simulink model "FSAC2021_V1"  (R2014a)
settings: Solver=FixedStepDiscrete  StartTime=0.0  StopTime=inf  FixedStep=0.0005  RelTol=1e-3
model workspace (MAT data in the model file):
  MCOS : class17 (value not decoded)
  MCOS : class17 (value not decoded)
  MCOS : class17 (value not decoded)
  MCOS : class17 (value not decoded)
  MCOS : class17 (value not decoded)
  MCOS : class17 (value not decoded)
  MCOS : class17 (value not decoded)
  MCOS : class17 (value not decoded)
  MCOS : class17 (value not decoded)
  MCOS : class17 (value not decoded)
  MCOS : class17 (value not decoded)
  MCOS : class17 (value not decoded)
  MCOS : class17 (value not decoded)
  MCOS : class17 (value not decoded)
  MCOS : class17 (value not decoded)
  MCOS : class17 (value not decoded)
  MCOS : class17 (value not decoded)
  MCOS : class17 (value not decoded)
  MCOS : class17 (value not decoded)
  BUZZER_START = 1
  MCOS : class17 (value not decoded)
  MCOS : class17 (value not decoded)
  MCOS : class17 (value not decoded)
  MCOS : class17 (value not decoded)
  MCOS : class17 (value not decoded)
  MCOS : class17 (value not decoded)
  MCOS : class17 (value not decoded)
  MCOS : class17 (value not decoded)
  MCOS : class17 (value not decoded)
  MCOS : class17 (value not decoded)
  MCOS : class17 (value not decoded)
  MCOS : class17 (value not decoded)
  MCOS : class17 (value not decoded)
  MCOS : class17 (value not decoded)
  MCOS : class17 (value not decoded)
  MCOS : class17 (value not decoded)
  MCOS : class17 (value not decoded)
  MCOS : class17 (value not decoded)
  MCOS : class17 (value not decoded)
  MCOS : class17 (value not decoded)
  MCOS : class17 (value not decoded)
  MCOS : class17 (value not decoded)
  MCOS : class17 (value not decoded)
  MCOS : class17 (value not decoded)
  MCOS : class17 (value not decoded)
  MCOS : class17 (value not decoded)
  MCOS : class17 (value not decoded)
  MCOS : class17 (value not decoded)
  MCOS : class17 (value not decoded)
  MCOS : class17 (value not decoded)
  MCOS : class17 (value not decoded)
  MCOS : class17 (value not decoded)
  MCOS : class17 (value not decoded)
  MCOS : class17 (value not decoded)
  MCOS : class17 (value not decoded)
  MCOS : class17 (value not decoded)
  MCOS : class17 (value not decoded)
  MCOS : class17 (value not decoded)
  Brake = 11
  MCOS : class17 (value not decoded)
  MCOS : class17 (value not decoded)
  MCOS : class17 (value not decoded)
  MCOS : class17 (value not decoded)
  MCOS : class17 (value not decoded)
  MCOS : class17 (value not decoded)
  MCOS : class17 (value not decoded)
  MCOS : class17 (value not decoded)
  Sensor_Acc_b = 101.85
  Sensor_Acc_k = -0.0185
  Str_Sen_Orig_Angle = -341
  MCOS : class17 (value not decoded)
  Tire_D = 0.47
  T = 0.05
libraries: simulink x189, ec55xxlib x135
(part 7 of 9)

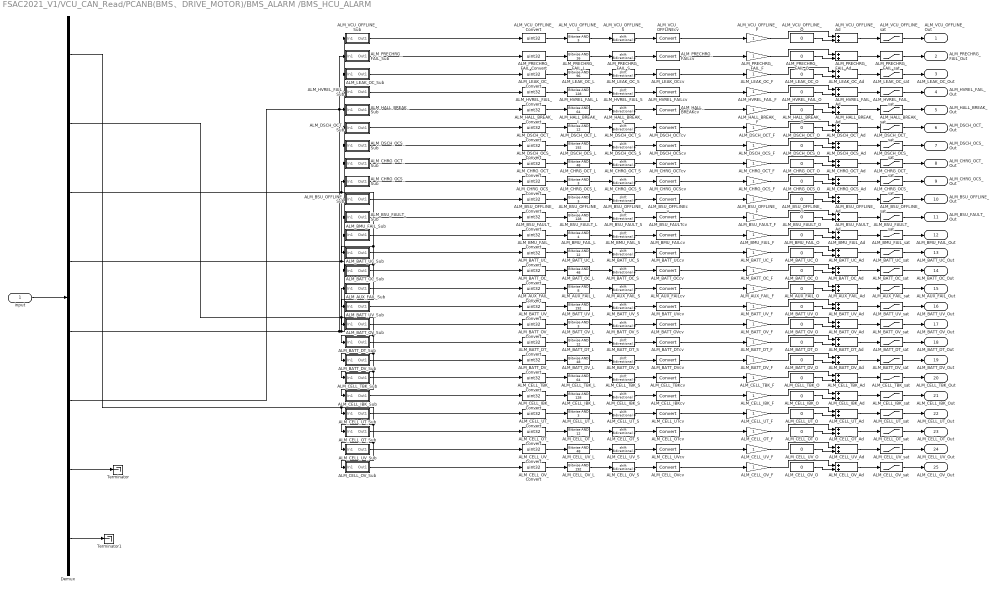
== system FSAC2021_V1/VCU_CAN_Read/PCANB(BMS、DRIVE_MOTOR)/BMS_ALARM /BMS_HCU_ALARM ==
  input : Inport
  ALM_AUX_FAIL_Ad : Sum
  ALM_AUX_FAIL_Convert : DataTypeConversion  OutDataTypeStr=uint32
  ALM_AUX_FAIL_F : Gain
  ALM_AUX_FAIL_L : simulink/Logic and Bit Operations/Bitwise Operator  logicop=AND  UseBitMask=on  BitMask=8  BitMaskRealWorld=Stored Integer
  ALM_AUX_FAIL_O : Constant  Value=0  OutDataTypeStr=single
  ALM_AUX_FAIL_S : ArithShift  BitShiftNumber=3
  ALM_AUX_FAIL_Sub : Subsystem
  ALM_AUX_FAIL_sat : Saturate  UpperLimit=1  LowerLimit=0
  ALM_AUX_FAILcv : DataTypeConversion
  ALM_BATT_DT_Ad : Sum
  ALM_BATT_DT_Convert : DataTypeConversion  OutDataTypeStr=uint32
  ALM_BATT_DT_F : Gain
  ALM_BATT_DT_L : simulink/Logic and Bit Operations/Bitwise Operator  logicop=AND  UseBitMask=on  BitMask=12  BitMaskRealWorld=Stored Integer
  ALM_BATT_DT_O : Constant  Value=0  OutDataTypeStr=single
  ALM_BATT_DT_S : ArithShift  BitShiftNumber=2
  ALM_BATT_DT_Sub : Subsystem
  ALM_BATT_DT_sat : Saturate  UpperLimit=3  LowerLimit=0
  ALM_BATT_DTcv : DataTypeConversion
  ALM_BATT_DV_Ad : Sum
  ALM_BATT_DV_Convert : DataTypeConversion  OutDataTypeStr=uint32
  ALM_BATT_DV_F : Gain
  ALM_BATT_DV_L : simulink/Logic and Bit Operations/Bitwise Operator  logicop=AND  UseBitMask=on  BitMask=48  BitMaskRealWorld=Stored Integer
  ALM_BATT_DV_O : Constant  Value=0  OutDataTypeStr=single
  ALM_BATT_DV_S : ArithShift  BitShiftNumber=4
  ALM_BATT_DV_Sub : Subsystem
  ALM_BATT_DV_sat : Saturate  UpperLimit=3  LowerLimit=0
  ALM_BATT_DVcv : DataTypeConversion
  ALM_BATT_OC_Ad : Sum
  ALM_BATT_OC_Convert : DataTypeConversion  OutDataTypeStr=uint32
  ALM_BATT_OC_F : Gain
  ALM_BATT_OC_L : simulink/Logic and Bit Operations/Bitwise Operator  logicop=AND  UseBitMask=on  BitMask=48  BitMaskRealWorld=Stored Integer
  ALM_BATT_OC_O : Constant  Value=0  OutDataTypeStr=single
  ALM_BATT_OC_S : ArithShift  BitShiftNumber=4
  ALM_BATT_OC_Sub : Subsystem
  ALM_BATT_OC_sat : Saturate  UpperLimit=3  LowerLimit=0
  ALM_BATT_OCcv : DataTypeConversion
  ALM_BATT_OV_Ad : Sum
  ALM_BATT_OV_Convert : DataTypeConversion  OutDataTypeStr=uint32
  ALM_BATT_OV_F : Gain
  ALM_BATT_OV_L : simulink/Logic and Bit Operations/Bitwise Operator  logicop=AND  UseBitMask=on  BitMask=3  BitMaskRealWorld=Stored Integer
  ALM_BATT_OV_O : Constant  Value=0  OutDataTypeStr=single
  ALM_BATT_OV_S : ArithShift
  ALM_BATT_OV_Sub : Subsystem
  ALM_BATT_OV_sat : Saturate  UpperLimit=3  LowerLimit=0
  ALM_BATT_OVcv : DataTypeConversion
  ALM_BATT_UC_Ad : Sum
  ALM_BATT_UC_Convert : DataTypeConversion  OutDataTypeStr=uint32
  ALM_BATT_UC_F : Gain
  ALM_BATT_UC_L : simulink/Logic and Bit Operations/Bitwise Operator  logicop=AND  UseBitMask=on  BitMask=12  BitMaskRealWorld=Stored Integer
  ALM_BATT_UC_O : Constant  Value=0  OutDataTypeStr=single
  ALM_BATT_UC_S : ArithShift  BitShiftNumber=2
  ALM_BATT_UC_Sub : Subsystem
  ALM_BATT_UC_sat : Saturate  UpperLimit=3  LowerLimit=0
  ALM_BATT_UCcv : DataTypeConversion
  ALM_BATT_UV_Ad : Sum
  ALM_BATT_UV_Convert : DataTypeConversion  OutDataTypeStr=uint32
  ALM_BATT_UV_F : Gain
  ALM_BATT_UV_L : simulink/Logic and Bit Operations/Bitwise Operator  logicop=AND  UseBitMask=on  BitMask=192  BitMaskRealWorld=Stored Integer
  ALM_BATT_UV_O : Constant  Value=0  OutDataTypeStr=single
  ALM_BATT_UV_S : ArithShift  BitShiftNumber=6
  ALM_BATT_UV_Sub : Subsystem
  ALM_BATT_UV_sat : Saturate  UpperLimit=3  LowerLimit=0
  ALM_BATT_UVcv : DataTypeConversion
  ALM_BMU_FAIL_Ad : Sum
  ALM_BMU_FAIL_Convert : DataTypeConversion  OutDataTypeStr=uint32
  ALM_BMU_FAIL_F : Gain
  ALM_BMU_FAIL_L : simulink/Logic and Bit Operations/Bitwise Operator  logicop=AND  UseBitMask=on  BitMask=4  BitMaskRealWorld=Stored Integer
  ALM_BMU_FAIL_O : Constant  Value=0  OutDataTypeStr=single
  ALM_BMU_FAIL_S : ArithShift  BitShiftNumber=2
  ALM_BMU_FAIL_Sub : Subsystem
  ALM_BMU_FAIL_sat : Saturate  UpperLimit=1  LowerLimit=0
  ALM_BMU_FAILcv : DataTypeConversion
  ALM_BSU_FAULT_Ad : Sum
  ALM_BSU_FAULT_Convert : DataTypeConversion  OutDataTypeStr=uint32
  ALM_BSU_FAULT_F : Gain
  ALM_BSU_FAULT_L : simulink/Logic and Bit Operations/Bitwise Operator  logicop=AND  UseBitMask=on  BitMask=128  BitMaskRealWorld=Stored Integer
  ALM_BSU_FAULT_O : Constant  Value=0  OutDataTypeStr=single
  ALM_BSU_FAULT_S : ArithShift  BitShiftNumber=7
  ALM_BSU_FAULT_Sub : Subsystem
  ALM_BSU_FAULT_sat : Saturate  UpperLimit=1  LowerLimit=0
  ALM_BSU_FAULTcv : DataTypeConversion
  ALM_BSU_OFFLINE_Ad : Sum
  ALM_BSU_OFFLINE_Convert : DataTypeConversion  OutDataTypeStr=uint32
  ALM_BSU_OFFLINE_F : Gain
  ALM_BSU_OFFLINE_L : simulink/Logic and Bit Operations/Bitwise Operator  logicop=AND  UseBitMask=on  BitMask=3  BitMaskRealWorld=Stored Integer
  ALM_BSU_OFFLINE_O : Constant  Value=0  OutDataTypeStr=single
  ALM_BSU_OFFLINE_S : ArithShift
  ALM_BSU_OFFLINE_Sub : Subsystem
  ALM_BSU_OFFLINE_sat : Saturate  UpperLimit=3  LowerLimit=0
  ALM_BSU_OFFLINEcv : DataTypeConversion
  ALM_CELL_IBK_Ad : Sum
  ALM_CELL_IBK_Convert : DataTypeConversion  OutDataTypeStr=uint32
  ALM_CELL_IBK_F : Gain
  ALM_CELL_IBK_L : simulink/Logic and Bit Operations/Bitwise Operator  logicop=AND  UseBitMask=on  BitMask=128  BitMaskRealWorld=Stored Integer
  ALM_CELL_IBK_O : Constant  Value=0  OutDataTypeStr=single
  ALM_CELL_IBK_S : ArithShift  BitShiftNumber=7
  ALM_CELL_IBK_Sub : Subsystem
  ALM_CELL_IBK_sat : Saturate  UpperLimit=1  LowerLimit=0
  ALM_CELL_IBKcv : DataTypeConversion
  ALM_CELL_OT_Ad : Sum
  ALM_CELL_OT_Convert : DataTypeConversion  OutDataTypeStr=uint32
  ALM_CELL_OT_F : Gain
  ALM_CELL_OT_L : simulink/Logic and Bit Operations/Bitwise Operator  logicop=AND  UseBitMask=on  BitMask=12  BitMaskRealWorld=Stored Integer
  ALM_CELL_OT_O : Constant  Value=0  OutDataTypeStr=single
  ALM_CELL_OT_S : ArithShift  BitShiftNumber=2
  ALM_CELL_OT_Sub : Subsystem
  ALM_CELL_OT_sat : Saturate  UpperLimit=3  LowerLimit=0
  ALM_CELL_OTcv : DataTypeConversion
  ALM_CELL_OV_Ad : Sum
  ALM_CELL_OV_Convert : DataTypeConversion  OutDataTypeStr=uint32
  ALM_CELL_OV_F : Gain
  ALM_CELL_OV_L : simulink/Logic and Bit Operations/Bitwise Operator  logicop=AND  UseBitMask=on  BitMask=192  BitMaskRealWorld=Stored Integer
  ALM_CELL_OV_O : Constant  Value=0  OutDataTypeStr=single
  ALM_CELL_OV_S : ArithShift  BitShiftNumber=6
  ALM_CELL_OV_Sub : Subsystem
  ALM_CELL_OV_sat : Saturate  UpperLimit=3  LowerLimit=0
  ALM_CELL_OVcv : DataTypeConversion
  ALM_CELL_TBK_Ad : Sum
  ALM_CELL_TBK_Convert : DataTypeConversion  OutDataTypeStr=uint32
  ALM_CELL_TBK_F : Gain
  ALM_CELL_TBK_L : simulink/Logic and Bit Operations/Bitwise Operator  logicop=AND  UseBitMask=on  BitMask=64  BitMaskRealWorld=Stored Integer
  ALM_CELL_TBK_O : Constant  Value=0  OutDataTypeStr=single
  ALM_CELL_TBK_S : ArithShift  BitShiftNumber=6
  ALM_CELL_TBK_Sub : Subsystem
  ALM_CELL_TBK_sat : Saturate  UpperLimit=1  LowerLimit=0
  ALM_CELL_TBKcv : DataTypeConversion
  ALM_CELL_UT_Ad : Sum
  ALM_CELL_UT_Convert : DataTypeConversion  OutDataTypeStr=uint32
  ALM_CELL_UT_F : Gain
  ALM_CELL_UT_L : simulink/Logic and Bit Operations/Bitwise Operator  logicop=AND  UseBitMask=on  BitMask=3  BitMaskRealWorld=Stored Integer
  ALM_CELL_UT_O : Constant  Value=0  OutDataTypeStr=single
  ALM_CELL_UT_S : ArithShift
  ALM_CELL_UT_Sub : Subsystem
  ALM_CELL_UT_sat : Saturate  UpperLimit=3  LowerLimit=0
  ALM_CELL_UTcv : DataTypeConversion
  ALM_CELL_UV_Ad : Sum
  ALM_CELL_UV_Convert : DataTypeConversion  OutDataTypeStr=uint32
  ALM_CELL_UV_F : Gain
  ALM_CELL_UV_L : simulink/Logic and Bit Operations/Bitwise Operator  logicop=AND  UseBitMask=on  BitMask=48  BitMaskRealWorld=Stored Integer
  ALM_CELL_UV_O : Constant  Value=0  OutDataTypeStr=single
  ALM_CELL_UV_S : ArithShift  BitShiftNumber=4
  ALM_CELL_UV_Sub : Subsystem
  ALM_CELL_UV_sat : Saturate  UpperLimit=3  LowerLimit=0
  ALM_CELL_UVcv : DataTypeConversion
  ALM_CHRG_OCS_Ad : Sum
  ALM_CHRG_OCS_Convert : DataTypeConversion  OutDataTypeStr=uint32
  ALM_CHRG_OCS_F : Gain
  ALM_CHRG_OCS_L : simulink/Logic and Bit Operations/Bitwise Operator  logicop=AND  UseBitMask=on  BitMask=3  BitMaskRealWorld=Stored Integer
  ALM_CHRG_OCS_O : Constant  Value=0  OutDataTypeStr=single
  ALM_CHRG_OCS_S : ArithShift
  ALM_CHRG_OCS_Sub : Subsystem
  ALM_CHRG_OCS_sat : Saturate  UpperLimit=3  LowerLimit=0
  ALM_CHRG_OCScv : DataTypeConversion
  ALM_CHRG_OCT_Ad : Sum
  ALM_CHRG_OCT_Convert : DataTypeConversion  OutDataTypeStr=uint32
  ALM_CHRG_OCT_F : Gain
  ALM_CHRG_OCT_L : simulink/Logic and Bit Operations/Bitwise Operator  logicop=AND  UseBitMask=on  BitMask=48  BitMaskRealWorld=Stored Integer
  ALM_CHRG_OCT_O : Constant  Value=0  OutDataTypeStr=single
  ALM_CHRG_OCT_S : ArithShift  BitShiftNumber=4
  ALM_CHRG_OCT_Sub : Subsystem
  ALM_CHRG_OCT_sat : Saturate  UpperLimit=3  LowerLimit=0
  ALM_CHRG_OCTcv : DataTypeConversion
  ALM_DSCH_OCS_Ad : Sum
  ALM_DSCH_OCS_Convert : DataTypeConversion  OutDataTypeStr=uint32
  ALM_DSCH_OCS_F : Gain
  ALM_DSCH_OCS_L : simulink/Logic and Bit Operations/Bitwise Operator  logicop=AND  UseBitMask=on  BitMask=192  BitMaskRealWorld=Stored Integer
  ALM_DSCH_OCS_O : Constant  Value=0  OutDataTypeStr=single
  ALM_DSCH_OCS_S : ArithShift  BitShiftNumber=6
  ALM_DSCH_OCS_Sub : Subsystem
  ALM_DSCH_OCS_sat : Saturate  UpperLimit=3  LowerLimit=0
  ALM_DSCH_OCScv : DataTypeConversion
  ALM_DSCH_OCT_Ad : Sum
  ALM_DSCH_OCT_Convert : DataTypeConversion  OutDataTypeStr=uint32
  ALM_DSCH_OCT_F : Gain
  ALM_DSCH_OCT_L : simulink/Logic and Bit Operations/Bitwise Operator  logicop=AND  UseBitMask=on  BitMask=12  BitMaskRealWorld=Stored Integer
  ALM_DSCH_OCT_O : Constant  Value=0  OutDataTypeStr=single
  ALM_DSCH_OCT_S : ArithShift  BitShiftNumber=2
  ALM_DSCH_OCT_Sub : Subsystem
  ALM_DSCH_OCT_sat : Saturate  UpperLimit=3  LowerLimit=0
  ALM_DSCH_OCTcv : DataTypeConversion
  ALM_HALL_BREAK_Ad : Sum
  ALM_HALL_BREAK_Convert : DataTypeConversion  OutDataTypeStr=uint32
  ALM_HALL_BREAK_F : Gain
  ALM_HALL_BREAK_L : simulink/Logic and Bit Operations/Bitwise Operator  logicop=AND  UseBitMask=on  BitMask=64  BitMaskRealWorld=Stored Integer
  ALM_HALL_BREAK_O : Constant  Value=0  OutDataTypeStr=single
  ALM_HALL_BREAK_S : ArithShift  BitShiftNumber=6
  ALM_HALL_BREAK_Sub : Subsystem
  ALM_HALL_BREAK_sat : Saturate  UpperLimit=1  LowerLimit=0
  ALM_HALL_BREAKcv : DataTypeConversion
  ALM_HVREL_FAIL_Ad : Sum
  ALM_HVREL_FAIL_Convert : DataTypeConversion  OutDataTypeStr=uint32
  ALM_HVREL_FAIL_F : Gain
  ALM_HVREL_FAIL_L : simulink/Logic and Bit Operations/Bitwise Operator  logicop=AND  UseBitMask=on  BitMask=128  BitMaskRealWorld=Stored Integer
  ALM_HVREL_FAIL_O : Constant  Value=0  OutDataTypeStr=single
  ALM_HVREL_FAIL_S : ArithShift  BitShiftNumber=7
  ALM_HVREL_FAIL_Sub : Subsystem
  ALM_HVREL_FAIL_sat : Saturate  UpperLimit=1  LowerLimit=0
  ALM_HVREL_FAILcv : DataTypeConversion
  ALM_LEAK_OC_Ad : Sum
  ALM_LEAK_OC_Convert : DataTypeConversion  OutDataTypeStr=uint32
  ALM_LEAK_OC_F : Gain
  ALM_LEAK_OC_L : simulink/Logic and Bit Operations/Bitwise Operator  logicop=AND  UseBitMask=on  BitMask=96  BitMaskRealWorld=Stored Integer
  ALM_LEAK_OC_O : Constant  Value=0  OutDataTypeStr=single
  ALM_LEAK_OC_S : ArithShift  BitShiftNumber=5
  ALM_LEAK_OC_Sub : Subsystem
  ALM_LEAK_OC_sat : Saturate  UpperLimit=3  LowerLimit=0
  ALM_LEAK_OCcv : DataTypeConversion
  ALM_PRECHRG_FAIL_Ad : Sum
  ALM_PRECHRG_FAIL_Convert : DataTypeConversion  OutDataTypeStr=uint32
  ALM_PRECHRG_FAIL_F : Gain
  ALM_PRECHRG_FAIL_L : simulink/Logic and Bit Operations/Bitwise Operator  logicop=AND  UseBitMask=on  BitMask=16  BitMaskRealWorld=Stored Integer
  ALM_PRECHRG_FAIL_O : Constant  Value=0  OutDataTypeStr=single
  ALM_PRECHRG_FAIL_S : ArithShift  BitShiftNumber=4
  ALM_PRECHRG_FAIL_Sub : Subsystem
  ALM_PRECHRG_FAIL_sat : Saturate  UpperLimit=1  LowerLimit=0
  ALM_PRECHRG_FAILcv : DataTypeConversion
  ALM_VCU_OFFLINE_Ad : Sum
  ALM_VCU_OFFLINE_Convert : DataTypeConversion  OutDataTypeStr=uint32
  ALM_VCU_OFFLINE_F : Gain
  ALM_VCU_OFFLINE_L : simulink/Logic and Bit Operations/Bitwise Operator  logicop=AND  UseBitMask=on  BitMask=3  BitMaskRealWorld=Stored Integer
  ALM_VCU_OFFLINE_O : Constant  Value=0  OutDataTypeStr=single
  ALM_VCU_OFFLINE_S : ArithShift
  ALM_VCU_OFFLINE_Sub : Subsystem
  ALM_VCU_OFFLINE_sat : Saturate  UpperLimit=3  LowerLimit=0
  ALM_VCU_OFFLINEcv : DataTypeConversion
  Demux : Demux  Outputs=8
  Terminator : Terminator
  Terminator1 : Terminator
  ALM_VCU_OFFLINE_Out : Outport
  ALM_PRECHRG_FAIL_Out : Outport  Port=2
  ALM_LEAK_OC_Out : Outport  Port=3
  ALM_HVREL_FAIL_Out : Outport  Port=4
  ALM_HALL_BREAK_Out : Outport  Port=5
  ALM_DSCH_OCT_Out : Outport  Port=6
  ALM_DSCH_OCS_Out : Outport  Port=7
  ALM_CHRG_OCT_Out : Outport  Port=8
  ALM_CHRG_OCS_Out : Outport  Port=9
  ALM_BSU_OFFLINE_Out : Outport  Port=10
  ALM_BSU_FAULT_Out : Outport  Port=11
  ALM_BMU_FAIL_Out : Outport  Port=12
  ALM_BATT_UC_Out : Outport  Port=13
  ALM_BATT_OC_Out : Outport  Port=14
  ALM_AUX_FAIL_Out : Outport  Port=15
  ALM_BATT_UV_Out : Outport  Port=16
  ALM_BATT_OV_Out : Outport  Port=17
  ALM_BATT_DT_Out : Outport  Port=18
  ALM_BATT_DV_Out : Outport  Port=19
  ALM_CELL_TBK_Out : Outport  Port=20
  ALM_CELL_IBK_Out : Outport  Port=21
  ALM_CELL_UT_Out : Outport  Port=22
  ALM_CELL_OT_Out : Outport  Port=23
  ALM_CELL_UV_Out : Outport  Port=24
  ALM_CELL_OV_Out : Outport  Port=25
  wires:
  ALM_VCU_OFFLINE_F/1 -> ALM_VCU_OFFLINE_Ad/1
  ALM_VCU_OFFLINE_O/1 -> ALM_VCU_OFFLINE_Ad/2
  ALM_VCU_OFFLINE_Ad/1 -> ALM_VCU_OFFLINE_sat/1
  ALM_VCU_OFFLINE_sat/1 -> ALM_VCU_OFFLINE_Out/1
  Demux/5 -> ALM_VCU_OFFLINE_Sub/1(In1), ALM_LEAK_OC_Sub/1(In1), ALM_BSU_FAULT_Sub/1(In1), ALM_BMU_FAIL_Sub/1(In1), ALM_AUX_FAIL_Sub/1(In1), ALM_PRECHRG_FAIL_Sub/1(In1)
  ALM_VCU_OFFLINE_Sub/1(Out1) -> ALM_VCU_OFFLINE_Convert/1
  ALM_VCU_OFFLINE_Convert/1 -> ALM_VCU_OFFLINE_L/1
  ALM_VCU_OFFLINE_L/1 -> ALM_VCU_OFFLINE_S/1
  ALM_VCU_OFFLINE_S/1 -> ALM_VCU_OFFLINEcv/1
  ALM_VCU_OFFLINEcv/1 -> ALM_VCU_OFFLINE_F/1
  ALM_PRECHRG_FAIL_F/1 -> ALM_PRECHRG_FAIL_Ad/1
  ALM_PRECHRG_FAIL_O/1 -> ALM_PRECHRG_FAIL_Ad/2
  ALM_PRECHRG_FAIL_Ad/1 -> ALM_PRECHRG_FAIL_sat/1
  ALM_PRECHRG_FAIL_sat/1 -> ALM_PRECHRG_FAIL_Out/1
  ALM_PRECHRG_FAIL_Sub/1(Out1) -> ALM_PRECHRG_FAIL_Convert/1
  ALM_PRECHRG_FAIL_Convert/1 -> ALM_PRECHRG_FAIL_L/1
  ALM_PRECHRG_FAIL_L/1 -> ALM_PRECHRG_FAIL_S/1
  ALM_PRECHRG_FAIL_S/1 -> ALM_PRECHRG_FAILcv/1
  ALM_PRECHRG_FAILcv/1 -> ALM_PRECHRG_FAIL_F/1
  ALM_LEAK_OC_F/1 -> ALM_LEAK_OC_Ad/1
  ALM_LEAK_OC_O/1 -> ALM_LEAK_OC_Ad/2
  ALM_LEAK_OC_Ad/1 -> ALM_LEAK_OC_sat/1
  ALM_LEAK_OC_sat/1 -> ALM_LEAK_OC_Out/1
  ALM_LEAK_OC_Sub/1(Out1) -> ALM_LEAK_OC_Convert/1
  ALM_LEAK_OC_Convert/1 -> ALM_LEAK_OC_L/1
  ALM_LEAK_OC_L/1 -> ALM_LEAK_OC_S/1
  ALM_LEAK_OC_S/1 -> ALM_LEAK_OCcv/1
  ALM_LEAK_OCcv/1 -> ALM_LEAK_OC_F/1
  ALM_HVREL_FAIL_F/1 -> ALM_HVREL_FAIL_Ad/1
  ALM_HVREL_FAIL_O/1 -> ALM_HVREL_FAIL_Ad/2
  ALM_HVREL_FAIL_Ad/1 -> ALM_HVREL_FAIL_sat/1
  ALM_HVREL_FAIL_sat/1 -> ALM_HVREL_FAIL_Out/1
  Demux/6 -> ALM_HVREL_FAIL_Sub/1(In1), ALM_HALL_BREAK_Sub/1(In1)
  ALM_HVREL_FAIL_Sub/1(Out1) -> ALM_HVREL_FAIL_Convert/1
  ALM_HVREL_FAIL_Convert/1 -> ALM_HVREL_FAIL_L/1
  ALM_HVREL_FAIL_L/1 -> ALM_HVREL_FAIL_S/1
  ALM_HVREL_FAIL_S/1 -> ALM_HVREL_FAILcv/1
  ALM_HVREL_FAILcv/1 -> ALM_HVREL_FAIL_F/1
  ALM_HALL_BREAK_F/1 -> ALM_HALL_BREAK_Ad/1
  ALM_HALL_BREAK_O/1 -> ALM_HALL_BREAK_Ad/2
  ALM_HALL_BREAK_Ad/1 -> ALM_HALL_BREAK_sat/1
  ALM_HALL_BREAK_sat/1 -> ALM_HALL_BREAK_Out/1
  ALM_HALL_BREAK_Sub/1(Out1) -> ALM_HALL_BREAK_Convert/1
  ALM_HALL_BREAK_Convert/1 -> ALM_HALL_BREAK_L/1
  ALM_HALL_BREAK_L/1 -> ALM_HALL_BREAK_S/1
  ALM_HALL_BREAK_S/1 -> ALM_HALL_BREAKcv/1
  ALM_HALL_BREAKcv/1 -> ALM_HALL_BREAK_F/1
  ALM_DSCH_OCT_F/1 -> ALM_DSCH_OCT_Ad/1
  ALM_DSCH_OCT_O/1 -> ALM_DSCH_OCT_Ad/2
  ALM_DSCH_OCT_Ad/1 -> ALM_DSCH_OCT_sat/1
  ALM_DSCH_OCT_sat/1 -> ALM_DSCH_OCT_Out/1
  Demux/4 -> ALM_DSCH_OCT_Sub/1(In1), ALM_DSCH_OCS_Sub/1(In1), ALM_CHRG_OCT_Sub/1(In1), ALM_BSU_OFFLINE_Sub/1(In1)
  ALM_DSCH_OCT_Sub/1(Out1) -> ALM_DSCH_OCT_Convert/1
  ALM_DSCH_OCT_Convert/1 -> ALM_DSCH_OCT_L/1
  ALM_DSCH_OCT_L/1 -> ALM_DSCH_OCT_S/1
  ALM_DSCH_OCT_S/1 -> ALM_DSCH_OCTcv/1
  ALM_DSCH_OCTcv/1 -> ALM_DSCH_OCT_F/1
  ALM_DSCH_OCS_F/1 -> ALM_DSCH_OCS_Ad/1
  ALM_DSCH_OCS_O/1 -> ALM_DSCH_OCS_Ad/2
  ALM_DSCH_OCS_Ad/1 -> ALM_DSCH_OCS_sat/1
  ALM_DSCH_OCS_sat/1 -> ALM_DSCH_OCS_Out/1
  ALM_DSCH_OCS_Sub/1(Out1) -> ALM_DSCH_OCS_Convert/1
  ALM_DSCH_OCS_Convert/1 -> ALM_DSCH_OCS_L/1
  ALM_DSCH_OCS_L/1 -> ALM_DSCH_OCS_S/1
  ALM_DSCH_OCS_S/1 -> ALM_DSCH_OCScv/1
  ALM_DSCH_OCScv/1 -> ALM_DSCH_OCS_F/1
  ALM_CHRG_OCT_F/1 -> ALM_CHRG_OCT_Ad/1
  ALM_CHRG_OCT_O/1 -> ALM_CHRG_OCT_Ad/2
  ALM_CHRG_OCT_Ad/1 -> ALM_CHRG_OCT_sat/1
  ALM_CHRG_OCT_sat/1 -> ALM_CHRG_OCT_Out/1
  ALM_CHRG_OCT_Sub/1(Out1) -> ALM_CHRG_OCT_Convert/1
  ALM_CHRG_OCT_Convert/1 -> ALM_CHRG_OCT_L/1
  ALM_CHRG_OCT_L/1 -> ALM_CHRG_OCT_S/1
  ALM_CHRG_OCT_S/1 -> ALM_CHRG_OCTcv/1
  ALM_CHRG_OCTcv/1 -> ALM_CHRG_OCT_F/1
  ALM_CHRG_OCS_F/1 -> ALM_CHRG_OCS_Ad/1
  ALM_CHRG_OCS_O/1 -> ALM_CHRG_OCS_Ad/2
  ALM_CHRG_OCS_Ad/1 -> ALM_CHRG_OCS_sat/1
  ALM_CHRG_OCS_sat/1 -> ALM_CHRG_OCS_Out/1
  Demux/3 -> ALM_BATT_OC_Sub/1(In1), ALM_BATT_UV_Sub/1(In1), ALM_BATT_UC_Sub/1(In1), ALM_CHRG_OCS_Sub/1(In1)
  ALM_CHRG_OCS_Sub/1(Out1) -> ALM_CHRG_OCS_Convert/1
  ALM_CHRG_OCS_Convert/1 -> ALM_CHRG_OCS_L/1
  ALM_CHRG_OCS_L/1 -> ALM_CHRG_OCS_S/1
  ALM_CHRG_OCS_S/1 -> ALM_CHRG_OCScv/1
  ALM_CHRG_OCScv/1 -> ALM_CHRG_OCS_F/1
  ALM_BSU_OFFLINE_F/1 -> ALM_BSU_OFFLINE_Ad/1
  ALM_BSU_OFFLINE_O/1 -> ALM_BSU_OFFLINE_Ad/2
  ALM_BSU_OFFLINE_Ad/1 -> ALM_BSU_OFFLINE_sat/1
  ALM_BSU_OFFLINE_sat/1 -> ALM_BSU_OFFLINE_Out/1
  ALM_BSU_OFFLINE_Sub/1(Out1) -> ALM_BSU_OFFLINE_Convert/1
  ALM_BSU_OFFLINE_Convert/1 -> ALM_BSU_OFFLINE_L/1
  ALM_BSU_OFFLINE_L/1 -> ALM_BSU_OFFLINE_S/1
  ALM_BSU_OFFLINE_S/1 -> ALM_BSU_OFFLINEcv/1
  ALM_BSU_OFFLINEcv/1 -> ALM_BSU_OFFLINE_F/1
  ALM_BSU_FAULT_F/1 -> ALM_BSU_FAULT_Ad/1
  ALM_BSU_FAULT_O/1 -> ALM_BSU_FAULT_Ad/2
  ALM_BSU_FAULT_Ad/1 -> ALM_BSU_FAULT_sat/1
  ALM_BSU_FAULT_sat/1 -> ALM_BSU_FAULT_Out/1
  ALM_BSU_FAULT_Sub/1(Out1) -> ALM_BSU_FAULT_Convert/1
  ALM_BSU_FAULT_Convert/1 -> ALM_BSU_FAULT_L/1
  ALM_BSU_FAULT_L/1 -> ALM_BSU_FAULT_S/1
  ALM_BSU_FAULT_S/1 -> ALM_BSU_FAULTcv/1
  ALM_BSU_FAULTcv/1 -> ALM_BSU_FAULT_F/1
  ALM_BMU_FAIL_F/1 -> ALM_BMU_FAIL_Ad/1
  ALM_BMU_FAIL_O/1 -> ALM_BMU_FAIL_Ad/2
  ALM_BMU_FAIL_Ad/1 -> ALM_BMU_FAIL_sat/1
  ALM_BMU_FAIL_sat/1 -> ALM_BMU_FAIL_Out/1
  ALM_BMU_FAIL_Sub/1(Out1) -> ALM_BMU_FAIL_Convert/1
  ALM_BMU_FAIL_Convert/1 -> ALM_BMU_FAIL_L/1
  ALM_BMU_FAIL_L/1 -> ALM_BMU_FAIL_S/1
  ALM_BMU_FAIL_S/1 -> ALM_BMU_FAILcv/1
  ALM_BMU_FAILcv/1 -> ALM_BMU_FAIL_F/1
  ALM_BATT_UC_F/1 -> ALM_BATT_UC_Ad/1
  ALM_BATT_UC_O/1 -> ALM_BATT_UC_Ad/2
  ALM_BATT_UC_Ad/1 -> ALM_BATT_UC_sat/1
  ALM_BATT_UC_sat/1 -> ALM_BATT_UC_Out/1
  ALM_BATT_UC_Sub/1(Out1) -> ALM_BATT_UC_Convert/1
  ALM_BATT_UC_Convert/1 -> ALM_BATT_UC_L/1
  ALM_BATT_UC_L/1 -> ALM_BATT_UC_S/1
  ALM_BATT_UC_S/1 -> ALM_BATT_UCcv/1
  ALM_BATT_UCcv/1 -> ALM_BATT_UC_F/1
  ALM_BATT_OC_F/1 -> ALM_BATT_OC_Ad/1
  ALM_BATT_OC_O/1 -> ALM_BATT_OC_Ad/2
  ALM_BATT_OC_Ad/1 -> ALM_BATT_OC_sat/1
  ALM_BATT_OC_sat/1 -> ALM_BATT_OC_Out/1
  ALM_BATT_OC_Sub/1(Out1) -> ALM_BATT_OC_Convert/1
  ALM_BATT_OC_Convert/1 -> ALM_BATT_OC_L/1
  ALM_BATT_OC_L/1 -> ALM_BATT_OC_S/1
  ALM_BATT_OC_S/1 -> ALM_BATT_OCcv/1
  ALM_BATT_OCcv/1 -> ALM_BATT_OC_F/1
  ALM_AUX_FAIL_F/1 -> ALM_AUX_FAIL_Ad/1
  ALM_AUX_FAIL_O/1 -> ALM_AUX_FAIL_Ad/2
  ALM_AUX_FAIL_Ad/1 -> ALM_AUX_FAIL_sat/1
  ALM_AUX_FAIL_sat/1 -> ALM_AUX_FAIL_Out/1
  ALM_AUX_FAIL_Sub/1(Out1) -> ALM_AUX_FAIL_Convert/1
  ALM_AUX_FAIL_Convert/1 -> ALM_AUX_FAIL_L/1
  ALM_AUX_FAIL_L/1 -> ALM_AUX_FAIL_S/1
  ALM_AUX_FAIL_S/1 -> ALM_AUX_FAILcv/1
  ALM_AUX_FAILcv/1 -> ALM_AUX_FAIL_F/1
  ALM_BATT_UV_F/1 -> ALM_BATT_UV_Ad/1
  ALM_BATT_UV_O/1 -> ALM_BATT_UV_Ad/2
  ALM_BATT_UV_Ad/1 -> ALM_BATT_UV_sat/1
  ALM_BATT_UV_sat/1 -> ALM_BATT_UV_Out/1
  ALM_BATT_UV_Sub/1(Out1) -> ALM_BATT_UV_Convert/1
  ALM_BATT_UV_Convert/1 -> ALM_BATT_UV_L/1
  ALM_BATT_UV_L/1 -> ALM_BATT_UV_S/1
  ALM_BATT_UV_S/1 -> ALM_BATT_UVcv/1
  ALM_BATT_UVcv/1 -> ALM_BATT_UV_F/1
  ALM_BATT_OV_F/1 -> ALM_BATT_OV_Ad/1
  ALM_BATT_OV_O/1 -> ALM_BATT_OV_Ad/2
  ALM_BATT_OV_Ad/1 -> ALM_BATT_OV_sat/1
  ALM_BATT_OV_sat/1 -> ALM_BATT_OV_Out/1
  Demux/2 -> ALM_CELL_TBK_Sub/1(In1), ALM_CELL_IBK_Sub/1(In1), ALM_BATT_DV_Sub/1(In1), ALM_BATT_DT_Sub/1(In1), ALM_BATT_OV_Sub/1(In1)
  ALM_BATT_OV_Sub/1(Out1) -> ALM_BATT_OV_Convert/1
  ALM_BATT_OV_Convert/1 -> ALM_BATT_OV_L/1
  ALM_BATT_OV_L/1 -> ALM_BATT_OV_S/1
  ALM_BATT_OV_S/1 -> ALM_BATT_OVcv/1
  ALM_BATT_OVcv/1 -> ALM_BATT_OV_F/1
  ALM_BATT_DT_F/1 -> ALM_BATT_DT_Ad/1
  ALM_BATT_DT_O/1 -> ALM_BATT_DT_Ad/2
  ALM_BATT_DT_Ad/1 -> ALM_BATT_DT_sat/1
  ALM_BATT_DT_sat/1 -> ALM_BATT_DT_Out/1
  ALM_BATT_DT_Sub/1(Out1) -> ALM_BATT_DT_Convert/1
  ALM_BATT_DT_Convert/1 -> ALM_BATT_DT_L/1
  ALM_BATT_DT_L/1 -> ALM_BATT_DT_S/1
  ALM_BATT_DT_S/1 -> ALM_BATT_DTcv/1
  ALM_BATT_DTcv/1 -> ALM_BATT_DT_F/1
  ALM_BATT_DV_F/1 -> ALM_BATT_DV_Ad/1
  ALM_BATT_DV_O/1 -> ALM_BATT_DV_Ad/2
  ALM_BATT_DV_Ad/1 -> ALM_BATT_DV_sat/1
  ALM_BATT_DV_sat/1 -> ALM_BATT_DV_Out/1
  ALM_BATT_DV_Sub/1(Out1) -> ALM_BATT_DV_Convert/1
  ALM_BATT_DV_Convert/1 -> ALM_BATT_DV_L/1
  ALM_BATT_DV_L/1 -> ALM_BATT_DV_S/1
  ALM_BATT_DV_S/1 -> ALM_BATT_DVcv/1
  ALM_BATT_DVcv/1 -> ALM_BATT_DV_F/1
  ALM_CELL_TBK_F/1 -> ALM_CELL_TBK_Ad/1
  ALM_CELL_TBK_O/1 -> ALM_CELL_TBK_Ad/2
  ALM_CELL_TBK_Ad/1 -> ALM_CELL_TBK_sat/1
  ALM_CELL_TBK_sat/1 -> ALM_CELL_TBK_Out/1
  ALM_CELL_TBK_Sub/1(Out1) -> ALM_CELL_TBK_Convert/1
  ALM_CELL_TBK_Convert/1 -> ALM_CELL_TBK_L/1
  ALM_CELL_TBK_L/1 -> ALM_CELL_TBK_S/1
  ALM_CELL_TBK_S/1 -> ALM_CELL_TBKcv/1
  ALM_CELL_TBKcv/1 -> ALM_CELL_TBK_F/1
  ALM_CELL_IBK_F/1 -> ALM_CELL_IBK_Ad/1
  ALM_CELL_IBK_O/1 -> ALM_CELL_IBK_Ad/2
  ALM_CELL_IBK_Ad/1 -> ALM_CELL_IBK_sat/1
  ALM_CELL_IBK_sat/1 -> ALM_CELL_IBK_Out/1
  ALM_CELL_IBK_Sub/1(Out1) -> ALM_CELL_IBK_Convert/1
  ALM_CELL_IBK_Convert/1 -> ALM_CELL_IBK_L/1
  ALM_CELL_IBK_L/1 -> ALM_CELL_IBK_S/1
  ALM_CELL_IBK_S/1 -> ALM_CELL_IBKcv/1
  ALM_CELL_IBKcv/1 -> ALM_CELL_IBK_F/1
  ALM_CELL_UT_F/1 -> ALM_CELL_UT_Ad/1
  ALM_CELL_UT_O/1 -> ALM_CELL_UT_Ad/2
  ALM_CELL_UT_Ad/1 -> ALM_CELL_UT_sat/1
  ALM_CELL_UT_sat/1 -> ALM_CELL_UT_Out/1
  Demux/1 -> ALM_CELL_UV_Sub/1(In1), ALM_CELL_OV_Sub/1(In1), ALM_CELL_OT_Sub/1(In1), ALM_CELL_UT_Sub/1(In1)
  ALM_CELL_UT_Sub/1(Out1) -> ALM_CELL_UT_Convert/1
  ALM_CELL_UT_Convert/1 -> ALM_CELL_UT_L/1
  ALM_CELL_UT_L/1 -> ALM_CELL_UT_S/1
  ALM_CELL_UT_S/1 -> ALM_CELL_UTcv/1
  ALM_CELL_UTcv/1 -> ALM_CELL_UT_F/1
  ALM_CELL_OT_F/1 -> ALM_CELL_OT_Ad/1
  ALM_CELL_OT_O/1 -> ALM_CELL_OT_Ad/2
  ALM_CELL_OT_Ad/1 -> ALM_CELL_OT_sat/1
  ALM_CELL_OT_sat/1 -> ALM_CELL_OT_Out/1
  ALM_CELL_OT_Sub/1(Out1) -> ALM_CELL_OT_Convert/1
  ALM_CELL_OT_Convert/1 -> ALM_CELL_OT_L/1
  ALM_CELL_OT_L/1 -> ALM_CELL_OT_S/1
  ALM_CELL_OT_S/1 -> ALM_CELL_OTcv/1
  ALM_CELL_OTcv/1 -> ALM_CELL_OT_F/1
  ALM_CELL_UV_F/1 -> ALM_CELL_UV_Ad/1
  ALM_CELL_UV_O/1 -> ALM_CELL_UV_Ad/2
  ALM_CELL_UV_Ad/1 -> ALM_CELL_UV_sat/1
  ALM_CELL_UV_sat/1 -> ALM_CELL_UV_Out/1
  ALM_CELL_UV_Sub/1(Out1) -> ALM_CELL_UV_Convert/1
  ALM_CELL_UV_Convert/1 -> ALM_CELL_UV_L/1
  ALM_CELL_UV_L/1 -> ALM_CELL_UV_S/1
  ALM_CELL_UV_S/1 -> ALM_CELL_UVcv/1
  ALM_CELL_UVcv/1 -> ALM_CELL_UV_F/1
  ALM_CELL_OV_F/1 -> ALM_CELL_OV_Ad/1
  ALM_CELL_OV_O/1 -> ALM_CELL_OV_Ad/2
  ALM_CELL_OV_Ad/1 -> ALM_CELL_OV_sat/1
  ALM_CELL_OV_sat/1 -> ALM_CELL_OV_Out/1
  ALM_CELL_OV_Sub/1(Out1) -> ALM_CELL_OV_Convert/1
  ALM_CELL_OV_Convert/1 -> ALM_CELL_OV_L/1
  ALM_CELL_OV_L/1 -> ALM_CELL_OV_S/1
  ALM_CELL_OV_S/1 -> ALM_CELL_OVcv/1
  ALM_CELL_OVcv/1 -> ALM_CELL_OV_F/1
  input/1 -> Demux/1
  Demux/7 -> Terminator/1
  Demux/8 -> Terminator1/1

== system FSAC2021_V1/VCU_CAN_Read/PCANB(BMS、DRIVE_MOTOR)/BMS_HCU_MAXT1/CoolingCtl_Sub ==
  In1 : Inport
  Out1 : Outport
  wires:
  In1/1 -> Out1/1

== system FSAC2021_V1/VCU_CAN_Read/PCANB(BMS、DRIVE_MOTOR)/BMS_HCU_MAXT1/HeatingCtl_Sub ==
  In1 : Inport
  Out1 : Outport
  wires:
  In1/1 -> Out1/1

== system FSAC2021_V1/VCU_CAN_Read/PCANB(BMS、DRIVE_MOTOR)/BMS_HCU_MAXT1/MaxTempNo_Sub ==
  In1 : Inport
  Out1 : Outport
  wires:
  In1/1 -> Out1/1

== system FSAC2021_V1/VCU_CAN_Read/PCANB(BMS、DRIVE_MOTOR)/BMS_HCU_MAXT1/MaxTemp_Sub ==
  In1 : Inport
  Out1 : Outport
  wires:
  In1/1 -> Out1/1

== system FSAC2021_V1/VCU_CAN_Read/PCANB(BMS、DRIVE_MOTOR)/BMS_HCU_MAXT1/MinTempNo_Sub ==
  In1 : Inport
  Out1 : Outport
  wires:
  In1/1 -> Out1/1

== system FSAC2021_V1/VCU_CAN_Read/PCANB(BMS、DRIVE_MOTOR)/BMS_HCU_MAXT1/MinTemp_Sub ==
  In1 : Inport
  Out1 : Outport
  wires:
  In1/1 -> Out1/1

== system FSAC2021_V1/VCU_CAN_Read/PCANB(BMS、DRIVE_MOTOR)/BMS_HCU_MAXV /BMS_HCU_MAXV ==
  input : Inport
  Demux : Demux  Outputs=8
  MaxCellVoltNo_Ad : Sum
  MaxCellVoltNo_Convert : DataTypeConversion  OutDataTypeStr=uint32
  MaxCellVoltNo_F : Gain
  MaxCellVoltNo_L : simulink/Logic and Bit Operations/Bitwise Operator  logicop=AND  UseBitMask=on  BitMask=255  BitMaskRealWorld=Stored Integer
  MaxCellVoltNo_O : Constant  Value=0  OutDataTypeStr=single
  MaxCellVoltNo_S : ArithShift
  MaxCellVoltNo_Sub : Subsystem
  MaxCellVoltNo_sat : Saturate  UpperLimit=255  LowerLimit=0
  MaxCellVoltNocv : DataTypeConversion
  MaxCellVolt_Ad : Sum
  MaxCellVolt_Convert : DataTypeConversion  OutDataTypeStr=uint32
  MaxCellVolt_F : Gain
  MaxCellVolt_L : simulink/Logic and Bit Operations/Bitwise Operator  logicop=AND  UseBitMask=on  BitMask=65535  BitMaskRealWorld=Stored Integer
  MaxCellVolt_O : Constant  Value=0  OutDataTypeStr=single
  MaxCellVolt_S : ArithShift
  MaxCellVolt_Sub : Subsystem
  MaxCellVolt_sat : Saturate  UpperLimit=5000  LowerLimit=0
  MaxCellVoltcv : DataTypeConversion
  MaxCellVoltinput1_Ad : Sum
  MaxCellVoltinput1_C : Constant  Value=256
  MaxCellVoltinput1_P : Product
  MinCellVoltNo_Ad : Sum
  MinCellVoltNo_Convert : DataTypeConversion  OutDataTypeStr=uint32
  MinCellVoltNo_F : Gain
  MinCellVoltNo_L : simulink/Logic and Bit Operations/Bitwise Operator  logicop=AND  UseBitMask=on  BitMask=255  BitMaskRealWorld=Stored Integer
  MinCellVoltNo_O : Constant  Value=0  OutDataTypeStr=single
  MinCellVoltNo_S : ArithShift
  MinCellVoltNo_Sub : Subsystem
  MinCellVoltNo_sat : Saturate  UpperLimit=255  LowerLimit=0
  MinCellVoltNocv : DataTypeConversion
  MinCellVolt_Ad : Sum
  MinCellVolt_Convert : DataTypeConversion  OutDataTypeStr=uint32
  MinCellVolt_F : Gain
  MinCellVolt_L : simulink/Logic and Bit Operations/Bitwise Operator  logicop=AND  UseBitMask=on  BitMask=65535  BitMaskRealWorld=Stored Integer
  MinCellVolt_O : Constant  Value=0  OutDataTypeStr=single
  MinCellVolt_S : ArithShift
  MinCellVolt_Sub : Subsystem
  MinCellVolt_sat : Saturate  UpperLimit=5000  LowerLimit=0
  MinCellVoltcv : DataTypeConversion
  MinCellVoltinput3_Ad : Sum
  MinCellVoltinput3_C : Constant  Value=256
  MinCellVoltinput3_P : Product
  Terminator : Terminator
  Terminator1 : Terminator
  MaxCellVoltNo_Out : Outport
  MinCellVoltNo_Out : Outport  Port=2
  MinCellVolt_Out : Outport  Port=3
  MaxCellVolt_Out : Outport  Port=4
  wires:
  MaxCellVoltNo_F/1 -> MaxCellVoltNo_Ad/1
  MaxCellVoltNo_O/1 -> MaxCellVoltNo_Ad/2
  MaxCellVoltNo_Ad/1 -> MaxCellVoltNo_sat/1
  MaxCellVoltNo_sat/1 -> MaxCellVoltNo_Out/1
  Demux/6 -> MaxCellVoltNo_Sub/1(In1)
  MaxCellVoltNo_Sub/1(Out1) -> MaxCellVoltNo_Convert/1
  MaxCellVoltNo_Convert/1 -> MaxCellVoltNo_L/1
  MaxCellVoltNo_L/1 -> MaxCellVoltNo_S/1
  MaxCellVoltNo_S/1 -> MaxCellVoltNocv/1
  MaxCellVoltNocv/1 -> MaxCellVoltNo_F/1
  MinCellVoltNo_F/1 -> MinCellVoltNo_Ad/1
  MinCellVoltNo_O/1 -> MinCellVoltNo_Ad/2
  MinCellVoltNo_Ad/1 -> MinCellVoltNo_sat/1
  MinCellVoltNo_sat/1 -> MinCellVoltNo_Out/1
  Demux/5 -> MinCellVoltNo_Sub/1(In1)
  MinCellVoltNo_Sub/1(Out1) -> MinCellVoltNo_Convert/1
  MinCellVoltNo_Convert/1 -> MinCellVoltNo_L/1
  MinCellVoltNo_L/1 -> MinCellVoltNo_S/1
  MinCellVoltNo_S/1 -> MinCellVoltNocv/1
  MinCellVoltNocv/1 -> MinCellVoltNo_F/1
  MinCellVolt_F/1 -> MinCellVolt_Ad/1
  MinCellVolt_O/1 -> MinCellVolt_Ad/2
  MinCellVolt_Ad/1 -> MinCellVolt_sat/1
  MinCellVolt_sat/1 -> MinCellVolt_Out/1
  Demux/3 -> MinCellVoltinput3_P/1
  MinCellVoltinput3_C/1 -> MinCellVoltinput3_P/2
  MinCellVoltinput3_P/1 -> MinCellVoltinput3_Ad/1
  Demux/4 -> MinCellVoltinput3_Ad/2
  MinCellVoltinput3_Ad/1 -> MinCellVolt_Sub/1(In1)
  MinCellVolt_Sub/1(Out1) -> MinCellVolt_Convert/1
  MinCellVolt_Convert/1 -> MinCellVolt_L/1
  MinCellVolt_L/1 -> MinCellVolt_S/1
  MinCellVolt_S/1 -> MinCellVoltcv/1
  MinCellVoltcv/1 -> MinCellVolt_F/1
  MaxCellVolt_F/1 -> MaxCellVolt_Ad/1
  MaxCellVolt_O/1 -> MaxCellVolt_Ad/2
  MaxCellVolt_Ad/1 -> MaxCellVolt_sat/1
  MaxCellVolt_sat/1 -> MaxCellVolt_Out/1
  Demux/1 -> MaxCellVoltinput1_P/1
  MaxCellVoltinput1_C/1 -> MaxCellVoltinput1_P/2
  MaxCellVoltinput1_P/1 -> MaxCellVoltinput1_Ad/1
  Demux/2 -> MaxCellVoltinput1_Ad/2
  MaxCellVoltinput1_Ad/1 -> MaxCellVolt_Sub/1(In1)
  MaxCellVolt_Sub/1(Out1) -> MaxCellVolt_Convert/1
  MaxCellVolt_Convert/1 -> MaxCellVolt_L/1
  MaxCellVolt_L/1 -> MaxCellVolt_S/1
  MaxCellVolt_S/1 -> MaxCellVoltcv/1
  MaxCellVoltcv/1 -> MaxCellVolt_F/1
  input/1 -> Demux/1
  Demux/7 -> Terminator/1
  Demux/8 -> Terminator1/1

== system FSAC2021_V1/VCU_CAN_Read/PCANB(BMS、DRIVE_MOTOR)/BMS_HCU_POWER /BMS_HCU_POWER ==
  input : Inport
  Demux : Demux  Outputs=8
  MaxChrCurtLimit_Ad : Sum
  MaxChrCurtLimit_Convert : DataTypeConversion  OutDataTypeStr=uint32
  MaxChrCurtLimit_F : Gain
  MaxChrCurtLimit_L : simulink/Logic and Bit Operations/Bitwise Operator  logicop=AND  UseBitMask=on  BitMask=65535  BitMaskRealWorld=Stored Integer
  MaxChrCurtLimit_O : Constant  Value=0  OutDataTypeStr=single
  MaxChrCurtLimit_S : ArithShift
  MaxChrCurtLimit_Sub : Subsystem
  MaxChrCurtLimit_sat : Saturate  UpperLimit=1000  LowerLimit=0
  MaxChrCurtLimitcv : DataTypeConversion
  MaxChrCurtLimitinput1_Ad : Sum
  MaxChrCurtLimitinput1_C : Constant  Value=256
  MaxChrCurtLimitinput1_P : Product
  MaxChrPowerLimit_Ad : Sum
  MaxChrPowerLimit_Convert : DataTypeConversion  OutDataTypeStr=uint32
  MaxChrPowerLimit_F : Gain  Gain=0.1
  MaxChrPowerLimit_L : simulink/Logic and Bit Operations/Bitwise Operator  logicop=AND  UseBitMask=on  BitMask=65535  BitMaskRealWorld=Stored Integer
  MaxChrPowerLimit_O : Constant  Value=0  OutDataTypeStr=single
  MaxChrPowerLimit_S : ArithShift
  MaxChrPowerLimit_Sub : Subsystem
  MaxChrPowerLimit_sat : Saturate  UpperLimit=300  LowerLimit=0
  MaxChrPowerLimitcv : DataTypeConversion
  MaxChrPowerLimitinput5_Ad : Sum
  MaxChrPowerLimitinput5_C : Constant  Value=256
  MaxChrPowerLimitinput5_P : Product
  MaxDisCurtLimit_Ad : Sum
  MaxDisCurtLimit_Convert : DataTypeConversion  OutDataTypeStr=uint32
  MaxDisCurtLimit_F : Gain
  MaxDisCurtLimit_L : simulink/Logic and Bit Operations/Bitwise Operator  logicop=AND  UseBitMask=on  BitMask=65535  BitMaskRealWorld=Stored Integer
  MaxDisCurtLimit_O : Constant  Value=0  OutDataTypeStr=single
  MaxDisCurtLimit_S : ArithShift
  MaxDisCurtLimit_Sub : Subsystem
  MaxDisCurtLimit_sat : Saturate  UpperLimit=1000  LowerLimit=0
  MaxDisCurtLimitcv : DataTypeConversion
  MaxDisCurtLimitinput3_Ad : Sum
  MaxDisCurtLimitinput3_C : Constant  Value=256
  MaxDisCurtLimitinput3_P : Product
  MaxDisPowerLimit_Ad : Sum
  MaxDisPowerLimit_Convert : DataTypeConversion  OutDataTypeStr=uint32
  MaxDisPowerLimit_F : Gain  Gain=0.1
  MaxDisPowerLimit_L : simulink/Logic and Bit Operations/Bitwise Operator  logicop=AND  UseBitMask=on  BitMask=65535  BitMaskRealWorld=Stored Integer
  MaxDisPowerLimit_O : Constant  Value=0  OutDataTypeStr=single
  MaxDisPowerLimit_S : ArithShift
  MaxDisPowerLimit_Sub : Subsystem
  MaxDisPowerLimit_sat : Saturate  UpperLimit=300  LowerLimit=0
  MaxDisPowerLimitcv : DataTypeConversion
  MaxDisPowerLimitinput7_Ad : Sum
  MaxDisPowerLimitinput7_C : Constant  Value=256
  MaxDisPowerLimitinput7_P : Product
  MaxDisPowerLimit_Out : Outport
  MaxChrPowerLimit_Out : Outport  Port=2
  MaxDisCurtLimit_Out : Outport  Port=3
  MaxChrCurtLimit_Out : Outport  Port=4
  wires:
  MaxDisPowerLimit_F/1 -> MaxDisPowerLimit_Ad/1
  MaxDisPowerLimit_O/1 -> MaxDisPowerLimit_Ad/2
  MaxDisPowerLimit_Ad/1 -> MaxDisPowerLimit_sat/1
  MaxDisPowerLimit_sat/1 -> MaxDisPowerLimit_Out/1
  Demux/7 -> MaxDisPowerLimitinput7_P/1
  MaxDisPowerLimitinput7_C/1 -> MaxDisPowerLimitinput7_P/2
  MaxDisPowerLimitinput7_P/1 -> MaxDisPowerLimitinput7_Ad/1
  Demux/8 -> MaxDisPowerLimitinput7_Ad/2
  MaxDisPowerLimitinput7_Ad/1 -> MaxDisPowerLimit_Sub/1(In1)
  MaxDisPowerLimit_Sub/1(Out1) -> MaxDisPowerLimit_Convert/1
  MaxDisPowerLimit_Convert/1 -> MaxDisPowerLimit_L/1
  MaxDisPowerLimit_L/1 -> MaxDisPowerLimit_S/1
  MaxDisPowerLimit_S/1 -> MaxDisPowerLimitcv/1
  MaxDisPowerLimitcv/1 -> MaxDisPowerLimit_F/1
  MaxChrPowerLimit_F/1 -> MaxChrPowerLimit_Ad/1
  MaxChrPowerLimit_O/1 -> MaxChrPowerLimit_Ad/2
  MaxChrPowerLimit_Ad/1 -> MaxChrPowerLimit_sat/1
  MaxChrPowerLimit_sat/1 -> MaxChrPowerLimit_Out/1
  Demux/5 -> MaxChrPowerLimitinput5_P/1
  MaxChrPowerLimitinput5_C/1 -> MaxChrPowerLimitinput5_P/2
  MaxChrPowerLimitinput5_P/1 -> MaxChrPowerLimitinput5_Ad/1
  Demux/6 -> MaxChrPowerLimitinput5_Ad/2
  MaxChrPowerLimitinput5_Ad/1 -> MaxChrPowerLimit_Sub/1(In1)
  MaxChrPowerLimit_Sub/1(Out1) -> MaxChrPowerLimit_Convert/1
  MaxChrPowerLimit_Convert/1 -> MaxChrPowerLimit_L/1
  MaxChrPowerLimit_L/1 -> MaxChrPowerLimit_S/1
  MaxChrPowerLimit_S/1 -> MaxChrPowerLimitcv/1
  MaxChrPowerLimitcv/1 -> MaxChrPowerLimit_F/1
  MaxDisCurtLimit_F/1 -> MaxDisCurtLimit_Ad/1
  MaxDisCurtLimit_O/1 -> MaxDisCurtLimit_Ad/2
  MaxDisCurtLimit_Ad/1 -> MaxDisCurtLimit_sat/1
  MaxDisCurtLimit_sat/1 -> MaxDisCurtLimit_Out/1
  Demux/3 -> MaxDisCurtLimitinput3_P/1
  MaxDisCurtLimitinput3_C/1 -> MaxDisCurtLimitinput3_P/2
  MaxDisCurtLimitinput3_P/1 -> MaxDisCurtLimitinput3_Ad/1
  Demux/4 -> MaxDisCurtLimitinput3_Ad/2
  MaxDisCurtLimitinput3_Ad/1 -> MaxDisCurtLimit_Sub/1(In1)
  MaxDisCurtLimit_Sub/1(Out1) -> MaxDisCurtLimit_Convert/1
  MaxDisCurtLimit_Convert/1 -> MaxDisCurtLimit_L/1
  MaxDisCurtLimit_L/1 -> MaxDisCurtLimit_S/1
  MaxDisCurtLimit_S/1 -> MaxDisCurtLimitcv/1
  MaxDisCurtLimitcv/1 -> MaxDisCurtLimit_F/1
  MaxChrCurtLimit_F/1 -> MaxChrCurtLimit_Ad/1
  MaxChrCurtLimit_O/1 -> MaxChrCurtLimit_Ad/2
  MaxChrCurtLimit_Ad/1 -> MaxChrCurtLimit_sat/1
  MaxChrCurtLimit_sat/1 -> MaxChrCurtLimit_Out/1
  Demux/1 -> MaxChrCurtLimitinput1_P/1
  MaxChrCurtLimitinput1_C/1 -> MaxChrCurtLimitinput1_P/2
  MaxChrCurtLimitinput1_P/1 -> MaxChrCurtLimitinput1_Ad/1
  Demux/2 -> MaxChrCurtLimitinput1_Ad/2
  MaxChrCurtLimitinput1_Ad/1 -> MaxChrCurtLimit_Sub/1(In1)
  MaxChrCurtLimit_Sub/1(Out1) -> MaxChrCurtLimit_Convert/1
  MaxChrCurtLimit_Convert/1 -> MaxChrCurtLimit_L/1
  MaxChrCurtLimit_L/1 -> MaxChrCurtLimit_S/1
  MaxChrCurtLimit_S/1 -> MaxChrCurtLimitcv/1
  MaxChrCurtLimitcv/1 -> MaxChrCurtLimit_F/1
  input/1 -> Demux/1

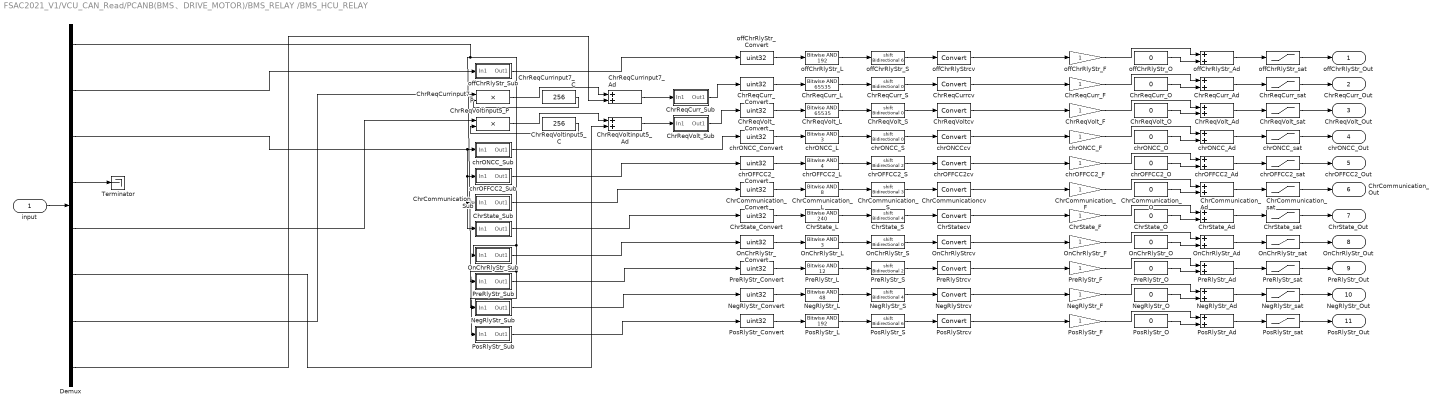
== system FSAC2021_V1/VCU_CAN_Read/PCANB(BMS、DRIVE_MOTOR)/BMS_RELAY /BMS_HCU_RELAY ==
  input : Inport
  ChrCommunication_Ad : Sum
  ChrCommunication_Convert : DataTypeConversion  OutDataTypeStr=uint32
  ChrCommunication_F : Gain
  ChrCommunication_L : simulink/Logic and Bit Operations/Bitwise Operator  logicop=AND  UseBitMask=on  BitMask=8  BitMaskRealWorld=Stored Integer
  ChrCommunication_O : Constant  Value=0  OutDataTypeStr=single
  ChrCommunication_S : ArithShift  BitShiftNumber=3
  ChrCommunication_Sub : Subsystem
  ChrCommunication_sat : Saturate  UpperLimit=1  LowerLimit=0
  ChrCommunicationcv : DataTypeConversion
  ChrReqCurr_Ad : Sum
  ChrReqCurr_Convert : DataTypeConversion  OutDataTypeStr=uint32
  ChrReqCurr_F : Gain
  ChrReqCurr_L : simulink/Logic and Bit Operations/Bitwise Operator  logicop=AND  UseBitMask=on  BitMask=65535  BitMaskRealWorld=Stored Integer
  ChrReqCurr_O : Constant  Value=0  OutDataTypeStr=single
  ChrReqCurr_S : ArithShift
  ChrReqCurr_Sub : Subsystem
  ChrReqCurr_sat : Saturate  UpperLimit=600  LowerLimit=0
  ChrReqCurrcv : DataTypeConversion
  ChrReqCurrinput7_Ad : Sum
  ChrReqCurrinput7_C : Constant  Value=256
  ChrReqCurrinput7_P : Product
  ChrReqVolt_Ad : Sum
  ChrReqVolt_Convert : DataTypeConversion  OutDataTypeStr=uint32
  ChrReqVolt_F : Gain
  ChrReqVolt_L : simulink/Logic and Bit Operations/Bitwise Operator  logicop=AND  UseBitMask=on  BitMask=65535  BitMaskRealWorld=Stored Integer
  ChrReqVolt_O : Constant  Value=0  OutDataTypeStr=single
  ChrReqVolt_S : ArithShift
  ChrReqVolt_Sub : Subsystem
  ChrReqVolt_sat : Saturate  UpperLimit=900  LowerLimit=0
  ChrReqVoltcv : DataTypeConversion
  ChrReqVoltinput5_Ad : Sum
  ChrReqVoltinput5_C : Constant  Value=256
  ChrReqVoltinput5_P : Product
  ChrState_Ad : Sum
  ChrState_Convert : DataTypeConversion  OutDataTypeStr=uint32
  ChrState_F : Gain
  ChrState_L : simulink/Logic and Bit Operations/Bitwise Operator  logicop=AND  UseBitMask=on  BitMask=240  BitMaskRealWorld=Stored Integer
  ChrState_O : Constant  Value=0  OutDataTypeStr=single
  ChrState_S : ArithShift  BitShiftNumber=4
  ChrState_Sub : Subsystem
  ChrState_sat : Saturate  UpperLimit=4  LowerLimit=0
  ChrStatecv : DataTypeConversion
  Demux : Demux  Outputs=8
  NegRlyStr_Ad : Sum
  NegRlyStr_Convert : DataTypeConversion  OutDataTypeStr=uint32
  NegRlyStr_F : Gain
  NegRlyStr_L : simulink/Logic and Bit Operations/Bitwise Operator  logicop=AND  UseBitMask=on  BitMask=48  BitMaskRealWorld=Stored Integer
  NegRlyStr_O : Constant  Value=0  OutDataTypeStr=single
  NegRlyStr_S : ArithShift  BitShiftNumber=4
  NegRlyStr_Sub : Subsystem
  NegRlyStr_sat : Saturate  UpperLimit=2  LowerLimit=0
  NegRlyStrcv : DataTypeConversion
  OnChrRlyStr_Ad : Sum
  OnChrRlyStr_Convert : DataTypeConversion  OutDataTypeStr=uint32
  OnChrRlyStr_F : Gain
  OnChrRlyStr_L : simulink/Logic and Bit Operations/Bitwise Operator  logicop=AND  UseBitMask=on  BitMask=3  BitMaskRealWorld=Stored Integer
  OnChrRlyStr_O : Constant  Value=0  OutDataTypeStr=single
  OnChrRlyStr_S : ArithShift
  OnChrRlyStr_Sub : Subsystem
  OnChrRlyStr_sat : Saturate  UpperLimit=2  LowerLimit=0
  OnChrRlyStrcv : DataTypeConversion
  PosRlyStr_Ad : Sum
  PosRlyStr_Convert : DataTypeConversion  OutDataTypeStr=uint32
  PosRlyStr_F : Gain
  PosRlyStr_L : simulink/Logic and Bit Operations/Bitwise Operator  logicop=AND  UseBitMask=on  BitMask=192  BitMaskRealWorld=Stored Integer
  PosRlyStr_O : Constant  Value=0  OutDataTypeStr=single
  PosRlyStr_S : ArithShift  BitShiftNumber=6
  PosRlyStr_Sub : Subsystem
  PosRlyStr_sat : Saturate  UpperLimit=2  LowerLimit=0
  PosRlyStrcv : DataTypeConversion
  PreRlyStr_Ad : Sum
  PreRlyStr_Convert : DataTypeConversion  OutDataTypeStr=uint32
  PreRlyStr_F : Gain
  PreRlyStr_L : simulink/Logic and Bit Operations/Bitwise Operator  logicop=AND  UseBitMask=on  BitMask=12  BitMaskRealWorld=Stored Integer
  PreRlyStr_O : Constant  Value=0  OutDataTypeStr=single
  PreRlyStr_S : ArithShift  BitShiftNumber=2
  PreRlyStr_Sub : Subsystem
  PreRlyStr_sat : Saturate  UpperLimit=2  LowerLimit=0
  PreRlyStrcv : DataTypeConversion
  Terminator : Terminator
  chrOFFCC2_Ad : Sum
  chrOFFCC2_Convert : DataTypeConversion  OutDataTypeStr=uint32
  chrOFFCC2_F : Gain
  chrOFFCC2_L : simulink/Logic and Bit Operations/Bitwise Operator  logicop=AND  UseBitMask=on  BitMask=4  BitMaskRealWorld=Stored Integer
  chrOFFCC2_O : Constant  Value=0  OutDataTypeStr=single
  chrOFFCC2_S : ArithShift  BitShiftNumber=2
  chrOFFCC2_Sub : Subsystem
  chrOFFCC2_sat : Saturate  UpperLimit=1  LowerLimit=0
  chrOFFCC2cv : DataTypeConversion
  chrONCC_Ad : Sum
  chrONCC_Convert : DataTypeConversion  OutDataTypeStr=uint32
  chrONCC_F : Gain
  chrONCC_L : simulink/Logic and Bit Operations/Bitwise Operator  logicop=AND  UseBitMask=on  BitMask=3  BitMaskRealWorld=Stored Integer
  chrONCC_O : Constant  Value=0  OutDataTypeStr=single
  chrONCC_S : ArithShift
  chrONCC_Sub : Subsystem
  chrONCC_sat : Saturate  UpperLimit=3  LowerLimit=0
  chrONCCcv : DataTypeConversion
  offChrRlyStr_Ad : Sum
  offChrRlyStr_Convert : DataTypeConversion  OutDataTypeStr=uint32
  offChrRlyStr_F : Gain
  offChrRlyStr_L : simulink/Logic and Bit Operations/Bitwise Operator  logicop=AND  UseBitMask=on  BitMask=192  BitMaskRealWorld=Stored Integer
  offChrRlyStr_O : Constant  Value=0  OutDataTypeStr=single
  offChrRlyStr_S : ArithShift  BitShiftNumber=6
  offChrRlyStr_Sub : Subsystem
  offChrRlyStr_sat : Saturate  UpperLimit=2  LowerLimit=0
  offChrRlyStrcv : DataTypeConversion
  offChrRlyStr_Out : Outport
  ChrReqCurr_Out : Outport  Port=2
  ChrReqVolt_Out : Outport  Port=3
  chrONCC_Out : Outport  Port=4
  chrOFFCC2_Out : Outport  Port=5
  ChrCommunication_Out : Outport  Port=6
  ChrState_Out : Outport  Port=7
  OnChrRlyStr_Out : Outport  Port=8
  PreRlyStr_Out : Outport  Port=9
  NegRlyStr_Out : Outport  Port=10
  PosRlyStr_Out : Outport  Port=11
  wires:
  offChrRlyStr_F/1 -> offChrRlyStr_Ad/1
  offChrRlyStr_O/1 -> offChrRlyStr_Ad/2
  offChrRlyStr_Ad/1 -> offChrRlyStr_sat/1
  offChrRlyStr_sat/1 -> offChrRlyStr_Out/1
  Demux/2 -> offChrRlyStr_Sub/1(In1)
  offChrRlyStr_Sub/1(Out1) -> offChrRlyStr_Convert/1
  offChrRlyStr_Convert/1 -> offChrRlyStr_L/1
  offChrRlyStr_L/1 -> offChrRlyStr_S/1
  offChrRlyStr_S/1 -> offChrRlyStrcv/1
  offChrRlyStrcv/1 -> offChrRlyStr_F/1
  ChrReqCurr_F/1 -> ChrReqCurr_Ad/1
  ChrReqCurr_O/1 -> ChrReqCurr_Ad/2
  ChrReqCurr_Ad/1 -> ChrReqCurr_sat/1
  ChrReqCurr_sat/1 -> ChrReqCurr_Out/1
  Demux/7 -> ChrReqCurrinput7_P/1
  ChrReqCurrinput7_C/1 -> ChrReqCurrinput7_P/2
  ChrReqCurrinput7_P/1 -> ChrReqCurrinput7_Ad/1
  Demux/8 -> ChrReqCurrinput7_Ad/2
  ChrReqCurrinput7_Ad/1 -> ChrReqCurr_Sub/1(In1)
  ChrReqCurr_Sub/1(Out1) -> ChrReqCurr_Convert/1
  ChrReqCurr_Convert/1 -> ChrReqCurr_L/1
  ChrReqCurr_L/1 -> ChrReqCurr_S/1
  ChrReqCurr_S/1 -> ChrReqCurrcv/1
  ChrReqCurrcv/1 -> ChrReqCurr_F/1
  ChrReqVolt_F/1 -> ChrReqVolt_Ad/1
  ChrReqVolt_O/1 -> ChrReqVolt_Ad/2
  ChrReqVolt_Ad/1 -> ChrReqVolt_sat/1
  ChrReqVolt_sat/1 -> ChrReqVolt_Out/1
  Demux/5 -> ChrReqVoltinput5_P/1
  ChrReqVoltinput5_C/1 -> ChrReqVoltinput5_P/2
  ChrReqVoltinput5_P/1 -> ChrReqVoltinput5_Ad/1
  Demux/6 -> ChrReqVoltinput5_Ad/2
  ChrReqVoltinput5_Ad/1 -> ChrReqVolt_Sub/1(In1)
  ChrReqVolt_Sub/1(Out1) -> ChrReqVolt_Convert/1
  ChrReqVolt_Convert/1 -> ChrReqVolt_L/1
  ChrReqVolt_L/1 -> ChrReqVolt_S/1
  ChrReqVolt_S/1 -> ChrReqVoltcv/1
  ChrReqVoltcv/1 -> ChrReqVolt_F/1
  chrONCC_F/1 -> chrONCC_Ad/1
  chrONCC_O/1 -> chrONCC_Ad/2
  chrONCC_Ad/1 -> chrONCC_sat/1
  chrONCC_sat/1 -> chrONCC_Out/1
  Demux/3 -> ChrCommunication_Sub/1(In1), ChrState_Sub/1(In1), chrOFFCC2_Sub/1(In1), chrONCC_Sub/1(In1)
  chrONCC_Sub/1(Out1) -> chrONCC_Convert/1
  chrONCC_Convert/1 -> chrONCC_L/1
  chrONCC_L/1 -> chrONCC_S/1
  chrONCC_S/1 -> chrONCCcv/1
  chrONCCcv/1 -> chrONCC_F/1
  chrOFFCC2_F/1 -> chrOFFCC2_Ad/1
  chrOFFCC2_O/1 -> chrOFFCC2_Ad/2
  chrOFFCC2_Ad/1 -> chrOFFCC2_sat/1
  chrOFFCC2_sat/1 -> chrOFFCC2_Out/1
  chrOFFCC2_Sub/1(Out1) -> chrOFFCC2_Convert/1
  chrOFFCC2_Convert/1 -> chrOFFCC2_L/1
  chrOFFCC2_L/1 -> chrOFFCC2_S/1
  chrOFFCC2_S/1 -> chrOFFCC2cv/1
  chrOFFCC2cv/1 -> chrOFFCC2_F/1
  ChrCommunication_F/1 -> ChrCommunication_Ad/1
  ChrCommunication_O/1 -> ChrCommunication_Ad/2
  ChrCommunication_Ad/1 -> ChrCommunication_sat/1
  ChrCommunication_sat/1 -> ChrCommunication_Out/1
  ChrCommunication_Sub/1(Out1) -> ChrCommunication_Convert/1
  ChrCommunication_Convert/1 -> ChrCommunication_L/1
  ChrCommunication_L/1 -> ChrCommunication_S/1
  ChrCommunication_S/1 -> ChrCommunicationcv/1
  ChrCommunicationcv/1 -> ChrCommunication_F/1
  ChrState_F/1 -> ChrState_Ad/1
  ChrState_O/1 -> ChrState_Ad/2
  ChrState_Ad/1 -> ChrState_sat/1
  ChrState_sat/1 -> ChrState_Out/1
  ChrState_Sub/1(Out1) -> ChrState_Convert/1
  ChrState_Convert/1 -> ChrState_L/1
  ChrState_L/1 -> ChrState_S/1
  ChrState_S/1 -> ChrStatecv/1
  ChrStatecv/1 -> ChrState_F/1
  OnChrRlyStr_F/1 -> OnChrRlyStr_Ad/1
  OnChrRlyStr_O/1 -> OnChrRlyStr_Ad/2
  OnChrRlyStr_Ad/1 -> OnChrRlyStr_sat/1
  OnChrRlyStr_sat/1 -> OnChrRlyStr_Out/1
  Demux/1 -> PreRlyStr_Sub/1(In1), NegRlyStr_Sub/1(In1), OnChrRlyStr_Sub/1(In1), PosRlyStr_Sub/1(In1)
  OnChrRlyStr_Sub/1(Out1) -> OnChrRlyStr_Convert/1
  OnChrRlyStr_Convert/1 -> OnChrRlyStr_L/1
  OnChrRlyStr_L/1 -> OnChrRlyStr_S/1
  OnChrRlyStr_S/1 -> OnChrRlyStrcv/1
  OnChrRlyStrcv/1 -> OnChrRlyStr_F/1
  PreRlyStr_F/1 -> PreRlyStr_Ad/1
  PreRlyStr_O/1 -> PreRlyStr_Ad/2
  PreRlyStr_Ad/1 -> PreRlyStr_sat/1
  PreRlyStr_sat/1 -> PreRlyStr_Out/1
  PreRlyStr_Sub/1(Out1) -> PreRlyStr_Convert/1
  PreRlyStr_Convert/1 -> PreRlyStr_L/1
  PreRlyStr_L/1 -> PreRlyStr_S/1
  PreRlyStr_S/1 -> PreRlyStrcv/1
  PreRlyStrcv/1 -> PreRlyStr_F/1
  NegRlyStr_F/1 -> NegRlyStr_Ad/1
  NegRlyStr_O/1 -> NegRlyStr_Ad/2
  NegRlyStr_Ad/1 -> NegRlyStr_sat/1
  NegRlyStr_sat/1 -> NegRlyStr_Out/1
  NegRlyStr_Sub/1(Out1) -> NegRlyStr_Convert/1
  NegRlyStr_Convert/1 -> NegRlyStr_L/1
  NegRlyStr_L/1 -> NegRlyStr_S/1
  NegRlyStr_S/1 -> NegRlyStrcv/1
  NegRlyStrcv/1 -> NegRlyStr_F/1
  PosRlyStr_F/1 -> PosRlyStr_Ad/1
  PosRlyStr_O/1 -> PosRlyStr_Ad/2
  PosRlyStr_Ad/1 -> PosRlyStr_sat/1
  PosRlyStr_sat/1 -> PosRlyStr_Out/1
  PosRlyStr_Sub/1(Out1) -> PosRlyStr_Convert/1
  PosRlyStr_Convert/1 -> PosRlyStr_L/1
  PosRlyStr_L/1 -> PosRlyStr_S/1
  PosRlyStr_S/1 -> PosRlyStrcv/1
  PosRlyStrcv/1 -> PosRlyStr_F/1
  input/1 -> Demux/1
  Demux/4 -> Terminator/1

== system FSAC2021_V1/VCU_CAN_Read/PCANB(BMS、DRIVE_MOTOR)/Heartt/assi_status_Sub ==
  In1 : Inport
  Out1 : Outport
  wires:
  In1/1 -> Out1/1

== system FSAC2021_V1/VCU_CAN_Read/PCANB(BMS、DRIVE_MOTOR)/MOTOR_CURRENT_SPEED/Motor_Currt_Speed_Sub ==
  In1 : Inport
  Out1 : Outport
  wires:
  In1/1 -> Out1/1
